simulink model "PruebaEncoders"  (R2023b)
settings: Solver=VariableStepAuto  StartTime=0.0  StopTime=inf  RelTol=1e-3
libraries: arduinosensorlib x2, simulink x1
settings Model: Creator=Diego  LastModifiedBy=Diego

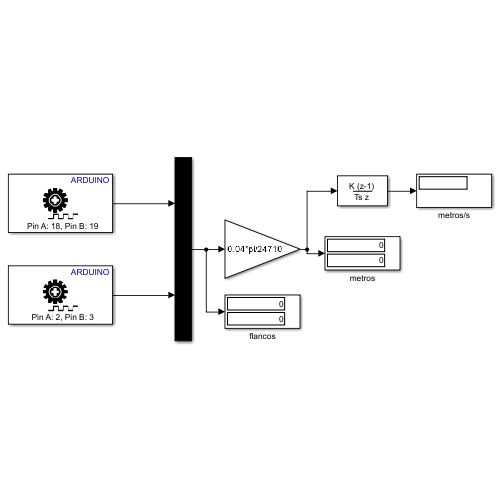
[thumbnail: Simulink's stored preview of the top-level diagram]
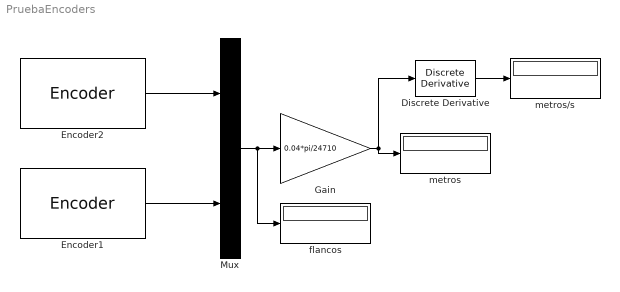
== system PruebaEncoders ==
  Discrete Derivative : simulink/Discrete/Discrete Derivative  gainval=1.0  ICPrevScaledInput=0.0  OutMin=[]  OutMax=[]  OutDataType=fixdt(1, 16)  OutScaling=2^-10  DoSatur=off
  Encoder1 : arduinosensorlib/Encoder  InputA=2  InputB=3  Mode=No reset  SampleTime=-1
  Encoder2 : arduinosensorlib/Encoder  InputA=18  InputB=19  Mode=No reset  SampleTime=-1
  Gain : Gain  Gain=0.04*pi/24710
  Mux : Mux  Inputs=2
  flancos : Display
  metros : Display
  metros/s : Display
  wires:
  Mux/1 -> flancos/1, Gain/1
  Encoder2/1 -> Mux/1
  Encoder1/1 -> Mux/2
  Gain/1 -> Discrete Derivative/1, metros/1
  Discrete Derivative/1 -> metros/s/1
